simulink model "Computer"  (R2019b)
settings: Solver=VariableStepAuto  StartTime=0.0  StopTime=inf  RelTol=1e-3
undefined symbols (not defined in the file): serial
libraries: instrumentlib x2
settings Model: EnablePacing=on  Creator=wuyuanyi  LastModifiedBy=wuyuanyi

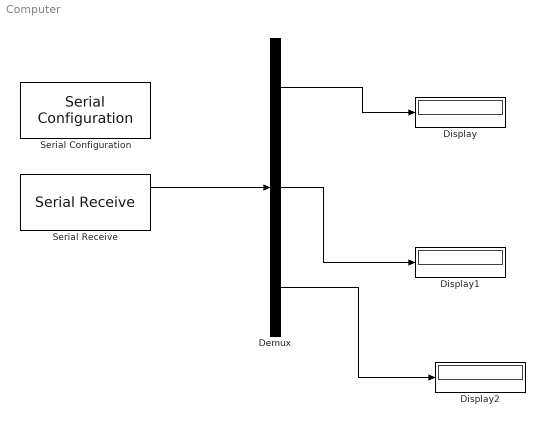
== system Computer ==
  Demux : Demux  Outputs=3
  Display : Display
  Display1 : Display
  Display2 : Display
  Serial Configuration : instrumentlib/Serial Configuration  Priority=-200000  ComPortMenu=/dev/ttyACM0  ComPort=/dev/ttyACM0  ObjConstructor=serial('/dev/ttyACM0');  BaudRate=9600  DataBits=8  Parity=none  StopBits=1  FlowControl=none  Timeout=10  ByteOrder=LittleEndian
  Serial Receive : instrumentlib/Serial Receive  ComPortMenu=/dev/ttyACM0  ComPort=/dev/ttyACM0  ObjConstructor=serial('/dev/ttyACM0');  Terminator=<none>  DataSize="[3  1]"  DataType=single  EnableBlockingMode=off  ActionDataUnavailable=Output last received value  CustomValue=0  SampleTime=1
  wires:
  Serial Receive/1 -> Demux/1
  Demux/1 -> Display/1
  Demux/2 -> Display1/1
  Demux/3 -> Display2/1
